simulink subsystem "VCM_main_ver3_0_0"  (R2021b)
settings: Solver=VariableStepAuto  StartTime=0.0  StopTime=10.0  RelTol=1e-3
undefined symbols (not defined in the file): g
libraries: simulink x46, dspswit3 x1, slpidlib x1
(part 4 of 5)

== system VCM_main_ver3_0_0/VDC/80kw_limitation/Power Limit_2/FL Power Culc ==
  FL Torque : Inport
  FL Actual Speed : Inport  Port=2
  2-D Lookup Table : Lookup_n-D  BreakpointsForDimension1="[1.3000    2.7000    5.4000    7.9000   10.4000   12.5000   14.4000   16.0000   17.4000   18.5000   19.6000]"  BreakpointsForDimension2="[ 500        1000        2000        3000        4000        6000       10000       12000       15000       19000]"  Table=|  InternalRulePriority=Speed  RndMeth=Simplest  InputSameDT=on
      | [ 0.6437    0.7133    0.7364    0.7470    0.7543    0.7657    0.7700    0.7708    0.7756    0.7814
      |     0.5842    0.7048    0.7757    0.8040    0.8201    0.8392    0.8516    0.8544    0.8597    0.8650
      |     0.4494    0.6081    0.7335    0.7882    0.8194    0.8543    0.8820    0.8888    0.8971    0.9044
      |     0.3559    0.5190    0.6702    0.7426    0.7854    0.8342    0.8758    0.8865    0.8984    0.9086
      |     0.2914    0.4478    0.6101    0.6941    0.7457    0.8062    0.8593    0.8758    0.8886    0.9016
      |     0.2417    0.3871    0.5522    0.6439    0.7024    0.7730    0.8373    0.8548    0.8737    0.8898
      |     0.2041    0.3371    0.5004    0.5965    0.6599    0.7388    0.8133    0.8342    0.8566    0.8759
      |     0.1731    0.2940    0.4510    0.5487    0.6155    0.7010    0.7856    0.8097    0.8356    0.8581
      |     0.1482    0.2575    0.4067    0.5041    0.5728    0.6634    0.7570    0.7840    0.8134    0.8271
      |     0.1281    0.2267    0.3672    0.4630    0.5325    0.6267    0.7277    0.7575    0.7902    0.7696
      |     0.1117    0.2005    0.3321    0.4251    0.4944    0.5909    0.6982    0.7306    0.6766    0.6928]
      settings: InputPortMap=u0,u1
  Divide : Product  Inputs=*/
  Gain : Gain  Gain=2*pi/60
  Product : Product
  Saturation : Saturate  UpperLimit=21  LowerLimit=0
  Saturation1 : Saturate  UpperLimit=19000  LowerLimit=0
  FL Power Consumption : Outport  VectorParamsAs1DForOutWhenUnconnected=off
  wires:
  Saturation1/1 -> Product/2, 2-D Lookup Table/2
  Saturation/1 -> Product/1, 2-D Lookup Table/1
  2-D Lookup Table/1 -> Divide/2  "FL Efficency"
  Product/1 -> Gain/1  "FL Motor Power"
  Divide/1 -> FL Power Consumption/1  "FL Power Consumption"
  FL Actual Speed/1 -> Saturation1/1
  FL Torque/1 -> Saturation/1
  Gain/1 -> Divide/1  "FL Motor Power_W"

== system VCM_main_ver3_0_0/VDC/80kw_limitation/Power Limit_2/FR Power Culc ==
  FR Torque : Inport
  FR Actual Speed : Inport  Port=2
  2-D Lookup Table : Lookup_n-D  BreakpointsForDimension1="[1.3000    2.7000    5.4000    7.9000   10.4000   12.5000   14.4000   16.0000   17.4000   18.5000   19.6000]"  BreakpointsForDimension2="[ 500        1000        2000        3000        4000        6000       10000       12000       15000       19000]"  Table=|  InternalRulePriority=Speed  RndMeth=Simplest  InputSameDT=on
      | [ 0.6437    0.7133    0.7364    0.7470    0.7543    0.7657    0.7700    0.7708    0.7756    0.7814
      |     0.5842    0.7048    0.7757    0.8040    0.8201    0.8392    0.8516    0.8544    0.8597    0.8650
      |     0.4494    0.6081    0.7335    0.7882    0.8194    0.8543    0.8820    0.8888    0.8971    0.9044
      |     0.3559    0.5190    0.6702    0.7426    0.7854    0.8342    0.8758    0.8865    0.8984    0.9086
      |     0.2914    0.4478    0.6101    0.6941    0.7457    0.8062    0.8593    0.8758    0.8886    0.9016
      |     0.2417    0.3871    0.5522    0.6439    0.7024    0.7730    0.8373    0.8548    0.8737    0.8898
      |     0.2041    0.3371    0.5004    0.5965    0.6599    0.7388    0.8133    0.8342    0.8566    0.8759
      |     0.1731    0.2940    0.4510    0.5487    0.6155    0.7010    0.7856    0.8097    0.8356    0.8581
      |     0.1482    0.2575    0.4067    0.5041    0.5728    0.6634    0.7570    0.7840    0.8134    0.8271
      |     0.1281    0.2267    0.3672    0.4630    0.5325    0.6267    0.7277    0.7575    0.7902    0.7696
      |     0.1117    0.2005    0.3321    0.4251    0.4944    0.5909    0.6982    0.7306    0.6766    0.6928]
      settings: InputPortMap=u0,u1
  Divide : Product  Inputs=*/
  Gain : Gain  Gain=2*pi/60
  Product : Product
  Saturation : Saturate  UpperLimit=21  LowerLimit=0
  Saturation1 : Saturate  UpperLimit=19000  LowerLimit=0
  Scope : Scope
  FR Power Consumption : Outport  VectorParamsAs1DForOutWhenUnconnected=off
  wires:
  Saturation1/1 -> Product/2, 2-D Lookup Table/2
  Saturation/1 -> Product/1, 2-D Lookup Table/1
  2-D Lookup Table/1 -> Divide/2  "FR Efficency"
  Product/1 -> Gain/1  "FR Motor Power"
  Divide/1 -> FR Power Consumption/1  "FR Power Consumption"
  FR Actual Speed/1 -> Saturation1/1
  FR Torque/1 -> Saturation/1
  Gain/1 -> Divide/1, Scope/1  "FR Motor Power_W"

== system VCM_main_ver3_0_0/VDC/80kw_limitation/Power Limit_2/RL Power Culc ==
  RL Torque : Inport
  RL Actual Speed : Inport  Port=2
  2-D Lookup Table : Lookup_n-D  BreakpointsForDimension1="[1.3000    2.7000    5.4000    7.9000   10.4000   12.5000   14.4000   16.0000   17.4000   18.5000   19.6000]"  BreakpointsForDimension2="[ 500        1000        2000        3000        4000        6000       10000       12000       15000       19000]"  Table=|  InternalRulePriority=Speed  RndMeth=Simplest  InputSameDT=on
      | [ 0.6437    0.7133    0.7364    0.7470    0.7543    0.7657    0.7700    0.7708    0.7756    0.7814
      |     0.5842    0.7048    0.7757    0.8040    0.8201    0.8392    0.8516    0.8544    0.8597    0.8650
      |     0.4494    0.6081    0.7335    0.7882    0.8194    0.8543    0.8820    0.8888    0.8971    0.9044
      |     0.3559    0.5190    0.6702    0.7426    0.7854    0.8342    0.8758    0.8865    0.8984    0.9086
      |     0.2914    0.4478    0.6101    0.6941    0.7457    0.8062    0.8593    0.8758    0.8886    0.9016
      |     0.2417    0.3871    0.5522    0.6439    0.7024    0.7730    0.8373    0.8548    0.8737    0.8898
      |     0.2041    0.3371    0.5004    0.5965    0.6599    0.7388    0.8133    0.8342    0.8566    0.8759
      |     0.1731    0.2940    0.4510    0.5487    0.6155    0.7010    0.7856    0.8097    0.8356    0.8581
      |     0.1482    0.2575    0.4067    0.5041    0.5728    0.6634    0.7570    0.7840    0.8134    0.8271
      |     0.1281    0.2267    0.3672    0.4630    0.5325    0.6267    0.7277    0.7575    0.7902    0.7696
      |     0.1117    0.2005    0.3321    0.4251    0.4944    0.5909    0.6982    0.7306    0.6766    0.6928]
      settings: InputPortMap=u0,u1
  Divide : Product  Inputs=*/
  Gain : Gain  Gain=2*pi/60
  Product : Product
  Saturation : Saturate  UpperLimit=21  LowerLimit=0
  Saturation1 : Saturate  UpperLimit=19000  LowerLimit=0
  RL Power Consumption : Outport  VectorParamsAs1DForOutWhenUnconnected=off
  wires:
  Saturation1/1 -> Product/2, 2-D Lookup Table/2
  Saturation/1 -> Product/1, 2-D Lookup Table/1
  2-D Lookup Table/1 -> Divide/2  "RL Efficency"
  Product/1 -> Gain/1  "RL Motor Power"
  Divide/1 -> RL Power Consumption/1  "RL Power Consumption"
  RL Actual Speed/1 -> Saturation1/1
  RL Torque/1 -> Saturation/1
  Gain/1 -> Divide/1  "RL Motor Power_W"

== system VCM_main_ver3_0_0/VDC/80kw_limitation/Power Limit_2/RR Power Culc ==
  RR Torque : Inport
  RR Actual Speed : Inport  Port=2
  2-D Lookup Table : Lookup_n-D  BreakpointsForDimension1="[1.3000    2.7000    5.4000    7.9000   10.4000   12.5000   14.4000   16.0000   17.4000   18.5000   19.6000]"  BreakpointsForDimension2="[ 500        1000        2000        3000        4000        6000       10000       12000       15000       19000]"  Table=|  InternalRulePriority=Speed  RndMeth=Simplest  InputSameDT=on
      | [ 0.6437    0.7133    0.7364    0.7470    0.7543    0.7657    0.7700    0.7708    0.7756    0.7814
      |     0.5842    0.7048    0.7757    0.8040    0.8201    0.8392    0.8516    0.8544    0.8597    0.8650
      |     0.4494    0.6081    0.7335    0.7882    0.8194    0.8543    0.8820    0.8888    0.8971    0.9044
      |     0.3559    0.5190    0.6702    0.7426    0.7854    0.8342    0.8758    0.8865    0.8984    0.9086
      |     0.2914    0.4478    0.6101    0.6941    0.7457    0.8062    0.8593    0.8758    0.8886    0.9016
      |     0.2417    0.3871    0.5522    0.6439    0.7024    0.7730    0.8373    0.8548    0.8737    0.8898
      |     0.2041    0.3371    0.5004    0.5965    0.6599    0.7388    0.8133    0.8342    0.8566    0.8759
      |     0.1731    0.2940    0.4510    0.5487    0.6155    0.7010    0.7856    0.8097    0.8356    0.8581
      |     0.1482    0.2575    0.4067    0.5041    0.5728    0.6634    0.7570    0.7840    0.8134    0.8271
      |     0.1281    0.2267    0.3672    0.4630    0.5325    0.6267    0.7277    0.7575    0.7902    0.7696
      |     0.1117    0.2005    0.3321    0.4251    0.4944    0.5909    0.6982    0.7306    0.6766    0.6928]
      settings: InputPortMap=u0,u1
  Divide : Product  Inputs=*/
  Gain : Gain  Gain=2*pi/60
  Product : Product
  Saturation : Saturate  UpperLimit=21  LowerLimit=0
  Saturation1 : Saturate  UpperLimit=19000  LowerLimit=0
  RR Power Consumption : Outport  VectorParamsAs1DForOutWhenUnconnected=off
  wires:
  Saturation1/1 -> Product/2, 2-D Lookup Table/2
  Saturation/1 -> Product/1, 2-D Lookup Table/1
  2-D Lookup Table/1 -> Divide/2  "RR Efficency"
  Product/1 -> Gain/1  "RR Motor Power"
  Divide/1 -> RR Power Consumption/1  "RR Power Consumption"
  RR Actual Speed/1 -> Saturation1/1
  RR Torque/1 -> Saturation/1
  Gain/1 -> Divide/1  "RR Motor Power_W"

== system VCM_main_ver3_0_0/VDC/80kw_limitation/Power Limit_3/FL Power Culc ==
  FL Torque : Inport
  FL Actual Speed : Inport  Port=2
  2-D Lookup Table : Lookup_n-D  BreakpointsForDimension1="[1.3000    2.7000    5.4000    7.9000   10.4000   12.5000   14.4000   16.0000   17.4000   18.5000   19.6000]"  BreakpointsForDimension2="[ 500        1000        2000        3000        4000        6000       10000       12000       15000       19000]"  Table=|  InternalRulePriority=Speed  RndMeth=Simplest  InputSameDT=on
      | [ 0.6437    0.7133    0.7364    0.7470    0.7543    0.7657    0.7700    0.7708    0.7756    0.7814
      |     0.5842    0.7048    0.7757    0.8040    0.8201    0.8392    0.8516    0.8544    0.8597    0.8650
      |     0.4494    0.6081    0.7335    0.7882    0.8194    0.8543    0.8820    0.8888    0.8971    0.9044
      |     0.3559    0.5190    0.6702    0.7426    0.7854    0.8342    0.8758    0.8865    0.8984    0.9086
      |     0.2914    0.4478    0.6101    0.6941    0.7457    0.8062    0.8593    0.8758    0.8886    0.9016
      |     0.2417    0.3871    0.5522    0.6439    0.7024    0.7730    0.8373    0.8548    0.8737    0.8898
      |     0.2041    0.3371    0.5004    0.5965    0.6599    0.7388    0.8133    0.8342    0.8566    0.8759
      |     0.1731    0.2940    0.4510    0.5487    0.6155    0.7010    0.7856    0.8097    0.8356    0.8581
      |     0.1482    0.2575    0.4067    0.5041    0.5728    0.6634    0.7570    0.7840    0.8134    0.8271
      |     0.1281    0.2267    0.3672    0.4630    0.5325    0.6267    0.7277    0.7575    0.7902    0.7696
      |     0.1117    0.2005    0.3321    0.4251    0.4944    0.5909    0.6982    0.7306    0.6766    0.6928]
      settings: InputPortMap=u0,u1
  Divide : Product  Inputs=*/
  Gain : Gain  Gain=2*pi/60
  Product : Product
  Saturation : Saturate  UpperLimit=21  LowerLimit=0
  Saturation1 : Saturate  UpperLimit=19000  LowerLimit=0
  FL Power Consumption : Outport  VectorParamsAs1DForOutWhenUnconnected=off
  wires:
  Gain/1 -> Divide/1  "FL Motor Power_W"
  FL Torque/1 -> Saturation/1
  FL Actual Speed/1 -> Saturation1/1
  Divide/1 -> FL Power Consumption/1  "FL Power Consumption"
  Product/1 -> Gain/1  "FL Motor Power"
  2-D Lookup Table/1 -> Divide/2  "FL Efficency"
  Saturation/1 -> 2-D Lookup Table/1, Product/1
  Saturation1/1 -> 2-D Lookup Table/2, Product/2

== system VCM_main_ver3_0_0/VDC/80kw_limitation/Power Limit_3/FR Power Culc ==
  FR Torque : Inport
  FR Actual Speed : Inport  Port=2
  2-D Lookup Table : Lookup_n-D  BreakpointsForDimension1="[1.3000    2.7000    5.4000    7.9000   10.4000   12.5000   14.4000   16.0000   17.4000   18.5000   19.6000]"  BreakpointsForDimension2="[ 500        1000        2000        3000        4000        6000       10000       12000       15000       19000]"  Table=|  InternalRulePriority=Speed  RndMeth=Simplest  InputSameDT=on
      | [ 0.6437    0.7133    0.7364    0.7470    0.7543    0.7657    0.7700    0.7708    0.7756    0.7814
      |     0.5842    0.7048    0.7757    0.8040    0.8201    0.8392    0.8516    0.8544    0.8597    0.8650
      |     0.4494    0.6081    0.7335    0.7882    0.8194    0.8543    0.8820    0.8888    0.8971    0.9044
      |     0.3559    0.5190    0.6702    0.7426    0.7854    0.8342    0.8758    0.8865    0.8984    0.9086
      |     0.2914    0.4478    0.6101    0.6941    0.7457    0.8062    0.8593    0.8758    0.8886    0.9016
      |     0.2417    0.3871    0.5522    0.6439    0.7024    0.7730    0.8373    0.8548    0.8737    0.8898
      |     0.2041    0.3371    0.5004    0.5965    0.6599    0.7388    0.8133    0.8342    0.8566    0.8759
      |     0.1731    0.2940    0.4510    0.5487    0.6155    0.7010    0.7856    0.8097    0.8356    0.8581
      |     0.1482    0.2575    0.4067    0.5041    0.5728    0.6634    0.7570    0.7840    0.8134    0.8271
      |     0.1281    0.2267    0.3672    0.4630    0.5325    0.6267    0.7277    0.7575    0.7902    0.7696
      |     0.1117    0.2005    0.3321    0.4251    0.4944    0.5909    0.6982    0.7306    0.6766    0.6928]
      settings: InputPortMap=u0,u1
  Divide : Product  Inputs=*/
  Gain : Gain  Gain=2*pi/60
  Product : Product
  Saturation : Saturate  UpperLimit=21  LowerLimit=0
  Saturation1 : Saturate  UpperLimit=19000  LowerLimit=0
  Scope : Scope
  FR Power Consumption : Outport  VectorParamsAs1DForOutWhenUnconnected=off
  wires:
  Gain/1 -> Scope/1, Divide/1  "FR Motor Power_W"
  FR Torque/1 -> Saturation/1
  FR Actual Speed/1 -> Saturation1/1
  Divide/1 -> FR Power Consumption/1  "FR Power Consumption"
  Product/1 -> Gain/1  "FR Motor Power"
  2-D Lookup Table/1 -> Divide/2  "FR Efficency"
  Saturation/1 -> 2-D Lookup Table/1, Product/1
  Saturation1/1 -> 2-D Lookup Table/2, Product/2

== system VCM_main_ver3_0_0/VDC/80kw_limitation/Power Limit_3/RL Power Culc ==
  RL Torque : Inport
  RL Actual Speed : Inport  Port=2
  2-D Lookup Table : Lookup_n-D  BreakpointsForDimension1="[1.3000    2.7000    5.4000    7.9000   10.4000   12.5000   14.4000   16.0000   17.4000   18.5000   19.6000]"  BreakpointsForDimension2="[ 500        1000        2000        3000        4000        6000       10000       12000       15000       19000]"  Table=|  InternalRulePriority=Speed  RndMeth=Simplest  InputSameDT=on
      | [ 0.6437    0.7133    0.7364    0.7470    0.7543    0.7657    0.7700    0.7708    0.7756    0.7814
      |     0.5842    0.7048    0.7757    0.8040    0.8201    0.8392    0.8516    0.8544    0.8597    0.8650
      |     0.4494    0.6081    0.7335    0.7882    0.8194    0.8543    0.8820    0.8888    0.8971    0.9044
      |     0.3559    0.5190    0.6702    0.7426    0.7854    0.8342    0.8758    0.8865    0.8984    0.9086
      |     0.2914    0.4478    0.6101    0.6941    0.7457    0.8062    0.8593    0.8758    0.8886    0.9016
      |     0.2417    0.3871    0.5522    0.6439    0.7024    0.7730    0.8373    0.8548    0.8737    0.8898
      |     0.2041    0.3371    0.5004    0.5965    0.6599    0.7388    0.8133    0.8342    0.8566    0.8759
      |     0.1731    0.2940    0.4510    0.5487    0.6155    0.7010    0.7856    0.8097    0.8356    0.8581
      |     0.1482    0.2575    0.4067    0.5041    0.5728    0.6634    0.7570    0.7840    0.8134    0.8271
      |     0.1281    0.2267    0.3672    0.4630    0.5325    0.6267    0.7277    0.7575    0.7902    0.7696
      |     0.1117    0.2005    0.3321    0.4251    0.4944    0.5909    0.6982    0.7306    0.6766    0.6928]
      settings: InputPortMap=u0,u1
  Divide : Product  Inputs=*/
  Gain : Gain  Gain=2*pi/60
  Product : Product
  Saturation : Saturate  UpperLimit=21  LowerLimit=0
  Saturation1 : Saturate  UpperLimit=19000  LowerLimit=0
  RL Power Consumption : Outport  VectorParamsAs1DForOutWhenUnconnected=off
  wires:
  Gain/1 -> Divide/1  "RL Motor Power_W"
  RL Torque/1 -> Saturation/1
  RL Actual Speed/1 -> Saturation1/1
  Divide/1 -> RL Power Consumption/1  "RL Power Consumption"
  Product/1 -> Gain/1  "RL Motor Power"
  2-D Lookup Table/1 -> Divide/2  "RL Efficency"
  Saturation/1 -> 2-D Lookup Table/1, Product/1
  Saturation1/1 -> 2-D Lookup Table/2, Product/2

== system VCM_main_ver3_0_0/VDC/80kw_limitation/Power Limit_3/RR Power Culc ==
  RR Torque : Inport
  RR Actual Speed : Inport  Port=2
  2-D Lookup Table : Lookup_n-D  BreakpointsForDimension1="[1.3000    2.7000    5.4000    7.9000   10.4000   12.5000   14.4000   16.0000   17.4000   18.5000   19.6000]"  BreakpointsForDimension2="[ 500        1000        2000        3000        4000        6000       10000       12000       15000       19000]"  Table=|  InternalRulePriority=Speed  RndMeth=Simplest  InputSameDT=on
      | [ 0.6437    0.7133    0.7364    0.7470    0.7543    0.7657    0.7700    0.7708    0.7756    0.7814
      |     0.5842    0.7048    0.7757    0.8040    0.8201    0.8392    0.8516    0.8544    0.8597    0.8650
      |     0.4494    0.6081    0.7335    0.7882    0.8194    0.8543    0.8820    0.8888    0.8971    0.9044
      |     0.3559    0.5190    0.6702    0.7426    0.7854    0.8342    0.8758    0.8865    0.8984    0.9086
      |     0.2914    0.4478    0.6101    0.6941    0.7457    0.8062    0.8593    0.8758    0.8886    0.9016
      |     0.2417    0.3871    0.5522    0.6439    0.7024    0.7730    0.8373    0.8548    0.8737    0.8898
      |     0.2041    0.3371    0.5004    0.5965    0.6599    0.7388    0.8133    0.8342    0.8566    0.8759
      |     0.1731    0.2940    0.4510    0.5487    0.6155    0.7010    0.7856    0.8097    0.8356    0.8581
      |     0.1482    0.2575    0.4067    0.5041    0.5728    0.6634    0.7570    0.7840    0.8134    0.8271
      |     0.1281    0.2267    0.3672    0.4630    0.5325    0.6267    0.7277    0.7575    0.7902    0.7696
      |     0.1117    0.2005    0.3321    0.4251    0.4944    0.5909    0.6982    0.7306    0.6766    0.6928]
      settings: InputPortMap=u0,u1
  Divide : Product  Inputs=*/
  Gain : Gain  Gain=2*pi/60
  Product : Product
  Saturation : Saturate  UpperLimit=21  LowerLimit=0
  Saturation1 : Saturate  UpperLimit=19000  LowerLimit=0
  RR Power Consumption : Outport  VectorParamsAs1DForOutWhenUnconnected=off
  wires:
  Gain/1 -> Divide/1  "RR Motor Power_W"
  RR Torque/1 -> Saturation/1
  RR Actual Speed/1 -> Saturation1/1
  Divide/1 -> RR Power Consumption/1  "RR Power Consumption"
  Product/1 -> Gain/1  "RR Motor Power"
  2-D Lookup Table/1 -> Divide/2  "RR Efficency"
  Saturation/1 -> 2-D Lookup Table/1, Product/1
  Saturation1/1 -> 2-D Lookup Table/2, Product/2

== system VCM_main_ver3_0_0/VDC/80kw_limitation/Power Limit_4/FL Power Culc ==
  FL Torque : Inport
  FL Actual Speed : Inport  Port=2
  2-D Lookup Table : Lookup_n-D  BreakpointsForDimension1="[1.3000    2.7000    5.4000    7.9000   10.4000   12.5000   14.4000   16.0000   17.4000   18.5000   19.6000]"  BreakpointsForDimension2="[ 500        1000        2000        3000        4000        6000       10000       12000       15000       19000]"  Table=|  InternalRulePriority=Speed  RndMeth=Simplest  InputSameDT=on
      | [ 0.6437    0.7133    0.7364    0.7470    0.7543    0.7657    0.7700    0.7708    0.7756    0.7814
      |     0.5842    0.7048    0.7757    0.8040    0.8201    0.8392    0.8516    0.8544    0.8597    0.8650
      |     0.4494    0.6081    0.7335    0.7882    0.8194    0.8543    0.8820    0.8888    0.8971    0.9044
      |     0.3559    0.5190    0.6702    0.7426    0.7854    0.8342    0.8758    0.8865    0.8984    0.9086
      |     0.2914    0.4478    0.6101    0.6941    0.7457    0.8062    0.8593    0.8758    0.8886    0.9016
      |     0.2417    0.3871    0.5522    0.6439    0.7024    0.7730    0.8373    0.8548    0.8737    0.8898
      |     0.2041    0.3371    0.5004    0.5965    0.6599    0.7388    0.8133    0.8342    0.8566    0.8759
      |     0.1731    0.2940    0.4510    0.5487    0.6155    0.7010    0.7856    0.8097    0.8356    0.8581
      |     0.1482    0.2575    0.4067    0.5041    0.5728    0.6634    0.7570    0.7840    0.8134    0.8271
      |     0.1281    0.2267    0.3672    0.4630    0.5325    0.6267    0.7277    0.7575    0.7902    0.7696
      |     0.1117    0.2005    0.3321    0.4251    0.4944    0.5909    0.6982    0.7306    0.6766    0.6928]
      settings: InputPortMap=u0,u1
  Divide : Product  Inputs=*/
  Gain : Gain  Gain=2*pi/60
  Product : Product
  Saturation : Saturate  UpperLimit=21  LowerLimit=0
  Saturation1 : Saturate  UpperLimit=19000  LowerLimit=0
  FL Power Consumption : Outport  VectorParamsAs1DForOutWhenUnconnected=off
  wires:
  Saturation1/1 -> Product/2, 2-D Lookup Table/2
  Saturation/1 -> Product/1, 2-D Lookup Table/1
  2-D Lookup Table/1 -> Divide/2  "FL Efficency"
  Product/1 -> Gain/1  "FL Motor Power"
  Divide/1 -> FL Power Consumption/1  "FL Power Consumption"
  FL Actual Speed/1 -> Saturation1/1
  FL Torque/1 -> Saturation/1
  Gain/1 -> Divide/1  "FL Motor Power_W"

== system VCM_main_ver3_0_0/VDC/80kw_limitation/Power Limit_4/FR Power Culc ==
  FR Torque : Inport
  FR Actual Speed : Inport  Port=2
  2-D Lookup Table : Lookup_n-D  BreakpointsForDimension1="[1.3000    2.7000    5.4000    7.9000   10.4000   12.5000   14.4000   16.0000   17.4000   18.5000   19.6000]"  BreakpointsForDimension2="[ 500        1000        2000        3000        4000        6000       10000       12000       15000       19000]"  Table=|  InternalRulePriority=Speed  RndMeth=Simplest  InputSameDT=on
      | [ 0.6437    0.7133    0.7364    0.7470    0.7543    0.7657    0.7700    0.7708    0.7756    0.7814
      |     0.5842    0.7048    0.7757    0.8040    0.8201    0.8392    0.8516    0.8544    0.8597    0.8650
      |     0.4494    0.6081    0.7335    0.7882    0.8194    0.8543    0.8820    0.8888    0.8971    0.9044
      |     0.3559    0.5190    0.6702    0.7426    0.7854    0.8342    0.8758    0.8865    0.8984    0.9086
      |     0.2914    0.4478    0.6101    0.6941    0.7457    0.8062    0.8593    0.8758    0.8886    0.9016
      |     0.2417    0.3871    0.5522    0.6439    0.7024    0.7730    0.8373    0.8548    0.8737    0.8898
      |     0.2041    0.3371    0.5004    0.5965    0.6599    0.7388    0.8133    0.8342    0.8566    0.8759
      |     0.1731    0.2940    0.4510    0.5487    0.6155    0.7010    0.7856    0.8097    0.8356    0.8581
      |     0.1482    0.2575    0.4067    0.5041    0.5728    0.6634    0.7570    0.7840    0.8134    0.8271
      |     0.1281    0.2267    0.3672    0.4630    0.5325    0.6267    0.7277    0.7575    0.7902    0.7696
      |     0.1117    0.2005    0.3321    0.4251    0.4944    0.5909    0.6982    0.7306    0.6766    0.6928]
      settings: InputPortMap=u0,u1
  Divide : Product  Inputs=*/
  Gain : Gain  Gain=2*pi/60
  Product : Product
  Saturation : Saturate  UpperLimit=21  LowerLimit=0
  Saturation1 : Saturate  UpperLimit=19000  LowerLimit=0
  Scope : Scope
  FR Power Consumption : Outport  VectorParamsAs1DForOutWhenUnconnected=off
  wires:
  Saturation1/1 -> Product/2, 2-D Lookup Table/2
  Saturation/1 -> Product/1, 2-D Lookup Table/1
  2-D Lookup Table/1 -> Divide/2  "FR Efficency"
  Product/1 -> Gain/1  "FR Motor Power"
  Divide/1 -> FR Power Consumption/1  "FR Power Consumption"
  FR Actual Speed/1 -> Saturation1/1
  FR Torque/1 -> Saturation/1
  Gain/1 -> Divide/1, Scope/1  "FR Motor Power_W"

== system VCM_main_ver3_0_0/VDC/80kw_limitation/Power Limit_4/RL Power Culc ==
  RL Torque : Inport
  RL Actual Speed : Inport  Port=2
  2-D Lookup Table : Lookup_n-D  BreakpointsForDimension1="[1.3000    2.7000    5.4000    7.9000   10.4000   12.5000   14.4000   16.0000   17.4000   18.5000   19.6000]"  BreakpointsForDimension2="[ 500        1000        2000        3000        4000        6000       10000       12000       15000       19000]"  Table=|  InternalRulePriority=Speed  RndMeth=Simplest  InputSameDT=on
      | [ 0.6437    0.7133    0.7364    0.7470    0.7543    0.7657    0.7700    0.7708    0.7756    0.7814
      |     0.5842    0.7048    0.7757    0.8040    0.8201    0.8392    0.8516    0.8544    0.8597    0.8650
      |     0.4494    0.6081    0.7335    0.7882    0.8194    0.8543    0.8820    0.8888    0.8971    0.9044
      |     0.3559    0.5190    0.6702    0.7426    0.7854    0.8342    0.8758    0.8865    0.8984    0.9086
      |     0.2914    0.4478    0.6101    0.6941    0.7457    0.8062    0.8593    0.8758    0.8886    0.9016
      |     0.2417    0.3871    0.5522    0.6439    0.7024    0.7730    0.8373    0.8548    0.8737    0.8898
      |     0.2041    0.3371    0.5004    0.5965    0.6599    0.7388    0.8133    0.8342    0.8566    0.8759
      |     0.1731    0.2940    0.4510    0.5487    0.6155    0.7010    0.7856    0.8097    0.8356    0.8581
      |     0.1482    0.2575    0.4067    0.5041    0.5728    0.6634    0.7570    0.7840    0.8134    0.8271
      |     0.1281    0.2267    0.3672    0.4630    0.5325    0.6267    0.7277    0.7575    0.7902    0.7696
      |     0.1117    0.2005    0.3321    0.4251    0.4944    0.5909    0.6982    0.7306    0.6766    0.6928]
      settings: InputPortMap=u0,u1
  Divide : Product  Inputs=*/
  Gain : Gain  Gain=2*pi/60
  Product : Product
  Saturation : Saturate  UpperLimit=21  LowerLimit=0
  Saturation1 : Saturate  UpperLimit=19000  LowerLimit=0
  RL Power Consumption : Outport  VectorParamsAs1DForOutWhenUnconnected=off
  wires:
  Saturation1/1 -> Product/2, 2-D Lookup Table/2
  Saturation/1 -> Product/1, 2-D Lookup Table/1
  2-D Lookup Table/1 -> Divide/2  "RL Efficency"
  Product/1 -> Gain/1  "RL Motor Power"
  Divide/1 -> RL Power Consumption/1  "RL Power Consumption"
  RL Actual Speed/1 -> Saturation1/1
  RL Torque/1 -> Saturation/1
  Gain/1 -> Divide/1  "RL Motor Power_W"

== system VCM_main_ver3_0_0/VDC/80kw_limitation/Power Limit_4/RR Power Culc ==
  RR Torque : Inport
  RR Actual Speed : Inport  Port=2
  2-D Lookup Table : Lookup_n-D  BreakpointsForDimension1="[1.3000    2.7000    5.4000    7.9000   10.4000   12.5000   14.4000   16.0000   17.4000   18.5000   19.6000]"  BreakpointsForDimension2="[ 500        1000        2000        3000        4000        6000       10000       12000       15000       19000]"  Table=|  InternalRulePriority=Speed  RndMeth=Simplest  InputSameDT=on
      | [ 0.6437    0.7133    0.7364    0.7470    0.7543    0.7657    0.7700    0.7708    0.7756    0.7814
      |     0.5842    0.7048    0.7757    0.8040    0.8201    0.8392    0.8516    0.8544    0.8597    0.8650
      |     0.4494    0.6081    0.7335    0.7882    0.8194    0.8543    0.8820    0.8888    0.8971    0.9044
      |     0.3559    0.5190    0.6702    0.7426    0.7854    0.8342    0.8758    0.8865    0.8984    0.9086
      |     0.2914    0.4478    0.6101    0.6941    0.7457    0.8062    0.8593    0.8758    0.8886    0.9016
      |     0.2417    0.3871    0.5522    0.6439    0.7024    0.7730    0.8373    0.8548    0.8737    0.8898
      |     0.2041    0.3371    0.5004    0.5965    0.6599    0.7388    0.8133    0.8342    0.8566    0.8759
      |     0.1731    0.2940    0.4510    0.5487    0.6155    0.7010    0.7856    0.8097    0.8356    0.8581
      |     0.1482    0.2575    0.4067    0.5041    0.5728    0.6634    0.7570    0.7840    0.8134    0.8271
      |     0.1281    0.2267    0.3672    0.4630    0.5325    0.6267    0.7277    0.7575    0.7902    0.7696
      |     0.1117    0.2005    0.3321    0.4251    0.4944    0.5909    0.6982    0.7306    0.6766    0.6928]
      settings: InputPortMap=u0,u1
  Divide : Product  Inputs=*/
  Gain : Gain  Gain=2*pi/60
  Product : Product
  Saturation : Saturate  UpperLimit=21  LowerLimit=0
  Saturation1 : Saturate  UpperLimit=19000  LowerLimit=0
  RR Power Consumption : Outport  VectorParamsAs1DForOutWhenUnconnected=off
  wires:
  Saturation1/1 -> Product/2, 2-D Lookup Table/2
  Saturation/1 -> Product/1, 2-D Lookup Table/1
  2-D Lookup Table/1 -> Divide/2  "RR Efficency"
  Product/1 -> Gain/1  "RR Motor Power"
  Divide/1 -> RR Power Consumption/1  "RR Power Consumption"
  RR Actual Speed/1 -> Saturation1/1
  RR Torque/1 -> Saturation/1
  Gain/1 -> Divide/1  "RR Motor Power_W"

== system VCM_main_ver3_0_0/VDC/80kw_limitation/Power Limit_5/FL Power Culc ==
  FL Torque : Inport
  FL Actual Speed : Inport  Port=2
  2-D Lookup Table : Lookup_n-D  BreakpointsForDimension1="[1.3000    2.7000    5.4000    7.9000   10.4000   12.5000   14.4000   16.0000   17.4000   18.5000   19.6000]"  BreakpointsForDimension2="[ 500        1000        2000        3000        4000        6000       10000       12000       15000       19000]"  Table=|  InternalRulePriority=Speed  RndMeth=Simplest  InputSameDT=on
      | [ 0.6437    0.7133    0.7364    0.7470    0.7543    0.7657    0.7700    0.7708    0.7756    0.7814
      |     0.5842    0.7048    0.7757    0.8040    0.8201    0.8392    0.8516    0.8544    0.8597    0.8650
      |     0.4494    0.6081    0.7335    0.7882    0.8194    0.8543    0.8820    0.8888    0.8971    0.9044
      |     0.3559    0.5190    0.6702    0.7426    0.7854    0.8342    0.8758    0.8865    0.8984    0.9086
      |     0.2914    0.4478    0.6101    0.6941    0.7457    0.8062    0.8593    0.8758    0.8886    0.9016
      |     0.2417    0.3871    0.5522    0.6439    0.7024    0.7730    0.8373    0.8548    0.8737    0.8898
      |     0.2041    0.3371    0.5004    0.5965    0.6599    0.7388    0.8133    0.8342    0.8566    0.8759
      |     0.1731    0.2940    0.4510    0.5487    0.6155    0.7010    0.7856    0.8097    0.8356    0.8581
      |     0.1482    0.2575    0.4067    0.5041    0.5728    0.6634    0.7570    0.7840    0.8134    0.8271
      |     0.1281    0.2267    0.3672    0.4630    0.5325    0.6267    0.7277    0.7575    0.7902    0.7696
      |     0.1117    0.2005    0.3321    0.4251    0.4944    0.5909    0.6982    0.7306    0.6766    0.6928]
      settings: InputPortMap=u0,u1
  Divide : Product  Inputs=*/
  Gain : Gain  Gain=2*pi/60
  Product : Product
  Saturation : Saturate  UpperLimit=21  LowerLimit=0
  Saturation1 : Saturate  UpperLimit=19000  LowerLimit=0
  FL Power Consumption : Outport  VectorParamsAs1DForOutWhenUnconnected=off
  wires:
  Gain/1 -> Divide/1  "FL Motor Power_W"
  FL Torque/1 -> Saturation/1
  FL Actual Speed/1 -> Saturation1/1
  Divide/1 -> FL Power Consumption/1  "FL Power Consumption"
  Product/1 -> Gain/1  "FL Motor Power"
  2-D Lookup Table/1 -> Divide/2  "FL Efficency"
  Saturation/1 -> 2-D Lookup Table/1, Product/1
  Saturation1/1 -> 2-D Lookup Table/2, Product/2

== system VCM_main_ver3_0_0/VDC/80kw_limitation/Power Limit_5/FR Power Culc ==
  FR Torque : Inport
  FR Actual Speed : Inport  Port=2
  2-D Lookup Table : Lookup_n-D  BreakpointsForDimension1="[1.3000    2.7000    5.4000    7.9000   10.4000   12.5000   14.4000   16.0000   17.4000   18.5000   19.6000]"  BreakpointsForDimension2="[ 500        1000        2000        3000        4000        6000       10000       12000       15000       19000]"  Table=|  InternalRulePriority=Speed  RndMeth=Simplest  InputSameDT=on
      | [ 0.6437    0.7133    0.7364    0.7470    0.7543    0.7657    0.7700    0.7708    0.7756    0.7814
      |     0.5842    0.7048    0.7757    0.8040    0.8201    0.8392    0.8516    0.8544    0.8597    0.8650
      |     0.4494    0.6081    0.7335    0.7882    0.8194    0.8543    0.8820    0.8888    0.8971    0.9044
      |     0.3559    0.5190    0.6702    0.7426    0.7854    0.8342    0.8758    0.8865    0.8984    0.9086
      |     0.2914    0.4478    0.6101    0.6941    0.7457    0.8062    0.8593    0.8758    0.8886    0.9016
      |     0.2417    0.3871    0.5522    0.6439    0.7024    0.7730    0.8373    0.8548    0.8737    0.8898
      |     0.2041    0.3371    0.5004    0.5965    0.6599    0.7388    0.8133    0.8342    0.8566    0.8759
      |     0.1731    0.2940    0.4510    0.5487    0.6155    0.7010    0.7856    0.8097    0.8356    0.8581
      |     0.1482    0.2575    0.4067    0.5041    0.5728    0.6634    0.7570    0.7840    0.8134    0.8271
      |     0.1281    0.2267    0.3672    0.4630    0.5325    0.6267    0.7277    0.7575    0.7902    0.7696
      |     0.1117    0.2005    0.3321    0.4251    0.4944    0.5909    0.6982    0.7306    0.6766    0.6928]
      settings: InputPortMap=u0,u1
  Divide : Product  Inputs=*/
  Gain : Gain  Gain=2*pi/60
  Product : Product
  Saturation : Saturate  UpperLimit=21  LowerLimit=0
  Saturation1 : Saturate  UpperLimit=19000  LowerLimit=0
  Scope : Scope
  FR Power Consumption : Outport  VectorParamsAs1DForOutWhenUnconnected=off
  wires:
  Gain/1 -> Scope/1, Divide/1  "FR Motor Power_W"
  FR Torque/1 -> Saturation/1
  FR Actual Speed/1 -> Saturation1/1
  Divide/1 -> FR Power Consumption/1  "FR Power Consumption"
  Product/1 -> Gain/1  "FR Motor Power"
  2-D Lookup Table/1 -> Divide/2  "FR Efficency"
  Saturation/1 -> 2-D Lookup Table/1, Product/1
  Saturation1/1 -> 2-D Lookup Table/2, Product/2

== system VCM_main_ver3_0_0/VDC/80kw_limitation/Power Limit_5/RL Power Culc ==
  RL Torque : Inport
  RL Actual Speed : Inport  Port=2
  2-D Lookup Table : Lookup_n-D  BreakpointsForDimension1="[1.3000    2.7000    5.4000    7.9000   10.4000   12.5000   14.4000   16.0000   17.4000   18.5000   19.6000]"  BreakpointsForDimension2="[ 500        1000        2000        3000        4000        6000       10000       12000       15000       19000]"  Table=|  InternalRulePriority=Speed  RndMeth=Simplest  InputSameDT=on
      | [ 0.6437    0.7133    0.7364    0.7470    0.7543    0.7657    0.7700    0.7708    0.7756    0.7814
      |     0.5842    0.7048    0.7757    0.8040    0.8201    0.8392    0.8516    0.8544    0.8597    0.8650
      |     0.4494    0.6081    0.7335    0.7882    0.8194    0.8543    0.8820    0.8888    0.8971    0.9044
      |     0.3559    0.5190    0.6702    0.7426    0.7854    0.8342    0.8758    0.8865    0.8984    0.9086
      |     0.2914    0.4478    0.6101    0.6941    0.7457    0.8062    0.8593    0.8758    0.8886    0.9016
      |     0.2417    0.3871    0.5522    0.6439    0.7024    0.7730    0.8373    0.8548    0.8737    0.8898
      |     0.2041    0.3371    0.5004    0.5965    0.6599    0.7388    0.8133    0.8342    0.8566    0.8759
      |     0.1731    0.2940    0.4510    0.5487    0.6155    0.7010    0.7856    0.8097    0.8356    0.8581
      |     0.1482    0.2575    0.4067    0.5041    0.5728    0.6634    0.7570    0.7840    0.8134    0.8271
      |     0.1281    0.2267    0.3672    0.4630    0.5325    0.6267    0.7277    0.7575    0.7902    0.7696
      |     0.1117    0.2005    0.3321    0.4251    0.4944    0.5909    0.6982    0.7306    0.6766    0.6928]
      settings: InputPortMap=u0,u1
  Divide : Product  Inputs=*/
  Gain : Gain  Gain=2*pi/60
  Product : Product
  Saturation : Saturate  UpperLimit=21  LowerLimit=0
  Saturation1 : Saturate  UpperLimit=19000  LowerLimit=0
  RL Power Consumption : Outport  VectorParamsAs1DForOutWhenUnconnected=off
  wires:
  Gain/1 -> Divide/1  "RL Motor Power_W"
  RL Torque/1 -> Saturation/1
  RL Actual Speed/1 -> Saturation1/1
  Divide/1 -> RL Power Consumption/1  "RL Power Consumption"
  Product/1 -> Gain/1  "RL Motor Power"
  2-D Lookup Table/1 -> Divide/2  "RL Efficency"
  Saturation/1 -> 2-D Lookup Table/1, Product/1
  Saturation1/1 -> 2-D Lookup Table/2, Product/2

== system VCM_main_ver3_0_0/VDC/80kw_limitation/Power Limit_5/RR Power Culc ==
  RR Torque : Inport
  RR Actual Speed : Inport  Port=2
  2-D Lookup Table : Lookup_n-D  BreakpointsForDimension1="[1.3000    2.7000    5.4000    7.9000   10.4000   12.5000   14.4000   16.0000   17.4000   18.5000   19.6000]"  BreakpointsForDimension2="[ 500        1000        2000        3000        4000        6000       10000       12000       15000       19000]"  Table=|  InternalRulePriority=Speed  RndMeth=Simplest  InputSameDT=on
      | [ 0.6437    0.7133    0.7364    0.7470    0.7543    0.7657    0.7700    0.7708    0.7756    0.7814
      |     0.5842    0.7048    0.7757    0.8040    0.8201    0.8392    0.8516    0.8544    0.8597    0.8650
      |     0.4494    0.6081    0.7335    0.7882    0.8194    0.8543    0.8820    0.8888    0.8971    0.9044
      |     0.3559    0.5190    0.6702    0.7426    0.7854    0.8342    0.8758    0.8865    0.8984    0.9086
      |     0.2914    0.4478    0.6101    0.6941    0.7457    0.8062    0.8593    0.8758    0.8886    0.9016
      |     0.2417    0.3871    0.5522    0.6439    0.7024    0.7730    0.8373    0.8548    0.8737    0.8898
      |     0.2041    0.3371    0.5004    0.5965    0.6599    0.7388    0.8133    0.8342    0.8566    0.8759
      |     0.1731    0.2940    0.4510    0.5487    0.6155    0.7010    0.7856    0.8097    0.8356    0.8581
      |     0.1482    0.2575    0.4067    0.5041    0.5728    0.6634    0.7570    0.7840    0.8134    0.8271
      |     0.1281    0.2267    0.3672    0.4630    0.5325    0.6267    0.7277    0.7575    0.7902    0.7696
      |     0.1117    0.2005    0.3321    0.4251    0.4944    0.5909    0.6982    0.7306    0.6766    0.6928]
      settings: InputPortMap=u0,u1
  Divide : Product  Inputs=*/
  Gain : Gain  Gain=2*pi/60
  Product : Product
  Saturation : Saturate  UpperLimit=21  LowerLimit=0
  Saturation1 : Saturate  UpperLimit=19000  LowerLimit=0
  RR Power Consumption : Outport  VectorParamsAs1DForOutWhenUnconnected=off
  wires:
  Gain/1 -> Divide/1  "RR Motor Power_W"
  RR Torque/1 -> Saturation/1
  RR Actual Speed/1 -> Saturation1/1
  Divide/1 -> RR Power Consumption/1  "RR Power Consumption"
  Product/1 -> Gain/1  "RR Motor Power"
  2-D Lookup Table/1 -> Divide/2  "RR Efficency"
  Saturation/1 -> 2-D Lookup Table/1, Product/1
  Saturation1/1 -> 2-D Lookup Table/2, Product/2

== system VCM_main_ver3_0_0/VDC/80kw_limitation/Power Limit_last/80kmLimitation_@HighSpeed ==
  In4 : Inport
  torque : Inport  Port=2
  torque1 : Inport  Port=3
  torque2 : Inport  Port=4
  torque3 : Inport  Port=5
  Bus Selector2 : BusSelector  OutputSignals=MC_21.MC2_Actual speed value in 1/rpm,MC_41.MC4_Actual speed value in 1/rpm,MC_31.MC3_Actual speed value in 1/rpm,MC_11.MC1_Actual speed value in 1/rpm
  Compare To Constant{,1..3} (4 alike) : simulink/Logic and Bit Operations/Compare To Constant  relop=<=  const=19300  OutDataTypeStr=boolean
  Saturation{,1..3} (4 alike) : Saturate  UpperLimit=8.72  LowerLimit=-inf
  Switch{4..7} (4 alike) : Switch  Criteria=u2 > Threshold
  RRtrq : Outport  VectorParamsAs1DForOutWhenUnconnected=off
  RLtrq : Outport  Port=2  VectorParamsAs1DForOutWhenUnconnected=off
  FRtrq : Outport  Port=3  VectorParamsAs1DForOutWhenUnconnected=off
  FLtrq : Outport  Port=4  VectorParamsAs1DForOutWhenUnconnected=off
  wires:
  torque2/1 -> Switch6/1, Saturation2/1
  Switch7/1 -> FLtrq/1  "FLtrq"
  Compare To Constant1/1 -> Switch5/2
  Compare To Constant/1 -> Switch4/2
  Bus Selector2/2 -> Compare To Constant1/1  "<MC4_Actual speed value in 1/rpm>"
  In4/1 -> Bus Selector2/1
  Bus Selector2/3 -> Compare To Constant2/1  "<MC3_Actual speed value in 1/rpm>"
  Compare To Constant2/1 -> Switch6/2
  Bus Selector2/1 -> Compare To Constant/1  "<MC2_Actual speed value in 1/rpm>"
  Compare To Constant3/1 -> Switch7/2
  Bus Selector2/4 -> Compare To Constant3/1  "<MC1_Actual speed value in 1/rpm>"
  Switch5/1 -> RLtrq/1  "RLtrq"
  Switch4/1 -> RRtrq/1  "RRtrq"
  torque/1 -> Saturation/1, Switch4/1
  Switch6/1 -> FRtrq/1  "FRtrq"
  torque3/1 -> Saturation3/1, Switch7/1
  torque1/1 -> Saturation1/1, Switch5/1
  Saturation/1 -> Switch4/3
  Saturation1/1 -> Switch5/3
  Saturation2/1 -> Switch6/3
  Saturation3/1 -> Switch7/3

== system VCM_main_ver3_0_0/VDC/DYC/YawmomentCal/FB ==
  r_ref : Inport
  <GYRO_Z> : Inport  Port=2
  Add1 : Sum  Inputs=+-
  PID Controller : slpidlib/PID Controller  Controller=PID  Form=Parallel  TimeDomain=Continuous-time  UseExternalTs=off  SampleTime=-1  IntegratorMethod=Forward Euler  FilterMethod=Forward Euler  ControllerParametersSource=internal  P=220  I=0  D=0  UseFilter=on  N=100  TunerSelectOption=Transfer Function Based (PID Tuner App)  InitialConditionSource=internal  InitialConditionForIntegrator=0  InitialConditionForFilter=0  DifferentiatorICPrevScaledInput=0  ExternalReset=none  TrackingMode=off  Kt=1  LimitOutput=off  SatLimitsSource=internal  UpperSaturationLimit=inf  LowerSaturationLimit=-inf  LinearizeAsGain=on  AntiWindupMode=none  Kb=1  POutMin=[]  POutMax=[]  IOutMin=[]  IOutMax=[]  DOutMin=[]  DOutMax=[]  NOutMin=[]  NOutMax=[]  SumOutMin=[]  SumOutMax=[]  SaturationOutMin=[]  SaturationOutMax=[]  PParamMin=[]  PParamMax=[]  IParamMin=[]  IParamMax=[]  DParamMin=[]  DParamMax=[]  NParamMin=[]  NParamMax=[]  KbParamMin=[]  KbParamMax=[]  KtParamMin=[]  KtParamMax=[]  KbOutMin=[]  KbOutMax=[]  KtOutMin=[]  KtOutMax=[]  IntegratorOutMin=[]  IntegratorOutMax=[]  FilterOutMin=[]  FilterOutMax=[]  SumI1OutMin=[]  SumI1OutMax=[]  SumI2OutMin=[]  SumI2OutMax=[]  SumI3OutMin=[]  SumI3OutMax=[]  SumI4OutMin=[]  SumI4OutMax=[]  SumDOutMin=[]  SumDOutMax=[]  DifferentiatorOutMin=[]  DifferentiatorOutMax=[]  FilterDiffOutCoefMin=[]  FilterDiffOutCoefMax=[]  ReciprocalOutMin=[]  ReciprocalOutMax=[]  SumDenOutMin=[]  SumDenOutMax=[]  SumNumOutMin=[]  SumNumOutMax=[]  DivideOutMin=[]  DivideOutMax=[]  UdiffTsProdOutMin=[]  UdiffTsProdOutMax=[]  NTsProdOutMin=[]  NTsProdOutMax=[]  UintegralTsProdOutMin=[]  UintegralTsProdOutMax=[]  UngainTsProdOutMin=[]  UngainTsProdOutMax=[]  FilterDenConstantOutDataTypeStr=Inherit: Inherit via back propagation  FilterDenConstantOutMin=[]  FilterDenConstantOutMax=[]  PCopyOutDataTypeStr=Inherit: Inherit via back propagation  PCopyOutMin=[]  PCopyOutMax=[]  NCopyOutDataTypeStr=Inherit: Inherit via back propagation  NCopyOutMin=[]  NCopyOutMax=[]  IntegratorContinuousStateAttributes=''  IntegratorStateMustResolveToSignalObject=off  IntegratorRTWStateStorageClass=Auto  FilterContinuousStateAttributes=''  FilterStateMustResolveToSignalObject=off  FilterRTWStateStorageClass=Auto  ParallelPVariant=InternalParameters  IdealPVariant=Disabled  IVariant=InternalParameters  DVariant=InternalParameters  IntegratorVariant=Continuous  SatVariant=Disabled  AWVariant=Passthrough  PCopyVariant=Disabled  TRVariant=Disabled  FdbkBlocksVariant=Forward  IdealPFdbkVariant=Disabled  SatFdbkVariant=Disabled  DerivativeFilterVariant=ContFilter  NVariant=InternalParameters  NCopyVariant=Disabled  FilterICVariant=InternalICsFilter  IntegratorICVariant=InternalICs  ExternalResetVariant=Disabled  TRSumVariant=Passthrough  SumFdbkVariant=Disabled  SumVariant=Sum_PID  TsampFilterVariant=InternalTs  TsampNgainVariant=Passthrough  TsampIntegralVariant=Passthrough  ExternalSaturationOutDataTypeStr=Inherit: Same as second input
  Scope : Scope
  Scope1 : Scope
  Transfer Fcn1 : TransferFcn  Denominator=[0.03 1]
  y : Outport
  wires:
  Add1/1 -> Scope/1, PID Controller/1
  PID Controller/1 -> y/1
  <GYRO_Z>/1 -> Transfer Fcn1/1
  Transfer Fcn1/1 -> Add1/2
  r_ref/1 -> Add1/1, Scope1/1

== system VCM_main_ver3_0_0/VDC/DYC/YawmomentCal/FF_Gain ==
  v [m/s] : Inport
  In1 : Inport  Port=2
  1-D Lookup Table : Lookup_n-D  NumberOfTableDimensions=1  BreakpointsForDimension1=[0 20 40 60 80]  TableSource=Input port  Table=[1 2 3 2 9 8 7 6 5 4 3]'  InterpMethod=Cubic spline  ExtrapMethod=Cubic spline  InternalRulePriority=Speed  RndMeth=Simplest  InputSameDT=on
      settings: InputPortMap=u0,p221
  Divide : Product  Inputs=**
  FFGain_0km/h : Constant
  FFGain_20km/h : Constant
  FFGain_40km/h : Constant
  FFGain_60km/h : Constant
  FFGain_80km/h : Constant
  Gain_DYC_FF : Gain  Gain=265
  Saturation : Saturate  UpperLimit=120  LowerLimit=0
  Vector Concatenate : Concatenate  NumInputs=5
  m/s to km/h : Gain  Gain=3.6
  Out1 : Outport
  wires:
  FFGain_60km/h/1 -> Vector Concatenate/4
  In1/1 -> Gain_DYC_FF/1
  Saturation/1 -> 1-D Lookup Table/1
  FFGain_0km/h/1 -> Vector Concatenate/1
  m/s to km/h/1 -> Saturation/1  "v"
  FFGain_20km/h/1 -> Vector Concatenate/2
  v [m/s]/1 -> m/s to km/h/1
  Vector Concatenate/1 -> 1-D Lookup Table/2
  FFGain_40km/h/1 -> Vector Concatenate/3
  Divide/1 -> Out1/1
  FFGain_80km/h/1 -> Vector Concatenate/5
  1-D Lookup Table/1 -> Divide/2
  Gain_DYC_FF/1 -> Divide/1

== system VCM_main_ver3_0_0/VDC/DYC/YawmomentCal/FF_diff_Gain ==
  v [m/s] : Inport
  In2 : Inport  Port=2
  1-D Lookup Table : Lookup_n-D  NumberOfTableDimensions=1  BreakpointsForDimension1=[0 20 40 60 80]  TableSource=Input port  Table=[1 2 3 2 9 8 7 6 5 4 3]'  InterpMethod=Cubic spline  ExtrapMethod=Cubic spline  InternalRulePriority=Speed  RndMeth=Simplest  InputSameDT=on
      settings: InputPortMap=u0,p221
  Divide : Product  Inputs=**
  FF_diff_Gain : Gain  Gain=1/3
  FFdiffGain_0km/h : Constant
  FFdiffGain_20km/h : Constant
  FFdiffGain_40km/h : Constant
  FFdiffGain_60km/h : Constant
  FFdiffGain_80km/h : Constant
  I : Gain  Gain=112
  Saturation : Saturate  UpperLimit=120  LowerLimit=0
  Transfer Fcn2 : TransferFcn  Numerator=[1 0]  Denominator=[0.01 1]
  Vector Concatenate : Concatenate  NumInputs=5
  m/s to km/h : Gain  Gain=3.6
  Out1 : Outport
  wires:
  FF_diff_Gain/1 -> Divide/1
  m/s to km/h/1 -> Saturation/1  "v"
  FFdiffGain_40km/h/1 -> Vector Concatenate/3
  FFdiffGain_80km/h/1 -> Vector Concatenate/5
  I/1 -> FF_diff_Gain/1
  FFdiffGain_60km/h/1 -> Vector Concatenate/4
  Vector Concatenate/1 -> 1-D Lookup Table/2
  Saturation/1 -> 1-D Lookup Table/1
  FFdiffGain_20km/h/1 -> Vector Concatenate/2
  FFdiffGain_0km/h/1 -> Vector Concatenate/1
  1-D Lookup Table/1 -> Divide/2
  Transfer Fcn2/1 -> I/1
  In2/1 -> Transfer Fcn2/1
  Divide/1 -> Out1/1
  v [m/s]/1 -> m/s to km/h/1

== system VCM_main_ver3_0_0/VDC/DYC/YawmomentCal/Velocity Clc ==
  Sensor : Inport
  Add : Sum
  Bus Selector : BusSelector  OutputSignals=CAN_from_IMU_139.VELOCITY_X,CAN_from_IMU_139.VELOCITY_Y
  Sqrt : Sqrt  SaturateOnIntegerOverflow=on
  Square1 : Math  Operator=square  SaturateOnIntegerOverflow=on
  Square2 : Math  Operator=square  SaturateOnIntegerOverflow=on
  v [m/s] : Outport
  wires:
  Bus Selector/2 -> Square2/1  "<VELOCITY_Y>"
  Bus Selector/1 -> Square1/1  "<VELOCITY_X>"
  Add/1 -> Sqrt/1
  Square1/1 -> Add/1
  Sensor/1 -> Bus Selector/1
  Square2/1 -> Add/2
  Sqrt/1 -> v [m/s]/1  "v [m/s]"

== system VCM_main_ver3_0_0/VDC/DYC/YawmomentCal/δ to r_noDYC ==
  v [m/s] : Inport
  StabilityFactor : Inport  Port=2
  SteerAngle : Inport  Port=3
  Add4 : Sum
  Constant3 : Constant
  Divide : Product  Inputs=**
  Divide2 : Product  Inputs=*/
  Divide3 : Product  Inputs=**
  Gain6 : Gain  Gain=1/1.53
  Product5 : Product
  r_noDYC : Outport
  wires:
  SteerAngle/1 -> Divide/2
  Divide/1 -> r_noDYC/1
  v [m/s]/1 -> Product5/2, Product5/1, Divide2/1
  Gain6/1 -> Divide/1
  Add4/1 -> Divide2/2
  Constant3/1 -> Add4/1
  Divide3/1 -> Add4/2
  Product5/1 -> Divide3/1
  Divide2/1 -> Gain6/1
  StabilityFactor/1 -> Divide3/2

== system VCM_main_ver3_0_0/VDC/DYC/YawmomentCal/δ to r_ref ==
  v [m/s] : Inport
  StabilityFactor : Inport  Port=2
  SteerAngle : Inport  Port=3
  Add4 : Sum
  Constant3 : Constant
  Divide : Product  Inputs=**
  Divide2 : Product  Inputs=*/
  Divide3 : Product  Inputs=**
  Gain6 : Gain  Gain=1/1.53
  Product5 : Product
  r_ref : Outport
  wires:
  StabilityFactor/1 -> Divide3/2
  Divide2/1 -> Gain6/1
  Product5/1 -> Divide3/1
  Divide3/1 -> Add4/2
  Constant3/1 -> Add4/1
  Add4/1 -> Divide2/2
  Gain6/1 -> Divide/1
  v [m/s]/1 -> Product5/1, Product5/2, Divide2/1
  Divide/1 -> r_ref/1
  SteerAngle/1 -> Divide/2

== system VCM_main_ver3_0_0/VDC/Traction Control/FF/1//(1-SlipRate) ==
  note: OUT=IN*1/1-λ
  In : Inport
  SlipRate : Inport  Port=2
  Add : Sum  Inputs=+-
  Constant2 : Constant
  Divide : Product  Inputs=*/
  Out : Outport
  wires:
  Constant2/1 -> Add/1
  Add/1 -> Divide/2
  SlipRate/1 -> Add/2
  Divide/1 -> Out/1
  In/1 -> Divide/1

== system VCM_main_ver3_0_0/VDC/Traction Control/Front TargetSpeedClc_inBrake/toTargetspeed ==
  note: 1/1-λ
  In1 : Inport
  In2 : Inport  Port=2
  Add : Sum  Inputs=+-
  Constant2 : Constant
  Divide : Product  Inputs=*/
  Out1 : Outport
  wires:
  Constant2/1 -> Add/1
  Add/1 -> Divide/2
  In1/1 -> Add/2
  Divide/1 -> Out1/1
  In2/1 -> Divide/1

== system VCM_main_ver3_0_0/VDC/Traction Control/Rear TargetSpeedClc_inAcc/toTargetspeed ==
  note: 1/1-λ
  In1 : Inport
  y : Inport  Port=2
  Add : Sum  Inputs=+-
  Constant2 : Constant
  Divide : Product  Inputs=*/
  Out1 : Outport
  wires:
  Constant2/1 -> Add/1
  Add/1 -> Divide/2
  In1/1 -> Add/2
  Divide/1 -> Out1/1
  y/1 -> Divide/1

== system VCM_main_ver3_0_0/VDC/Traction Control/Rear TargetSpeedClc_inBrake/toTargetspeed ==
  note: 1/1-λ
  In1 : Inport
  In2 : Inport  Port=2
  Add : Sum  Inputs=+-
  Constant2 : Constant
  Divide : Product  Inputs=*/
  Out1 : Outport
  wires:
  Constant2/1 -> Add/1
  Add/1 -> Divide/2
  In1/1 -> Add/2
  Divide/1 -> Out1/1
  In2/1 -> Divide/1
